simulink model "Electrochmical_simulink"  (R2022a)
settings: Solver=VariableStepAuto  StartTime=0.0  StopTime=10.0  RelTol=1e-3
settings Model: Creator=Anupp  LastModifiedBy=Anupp

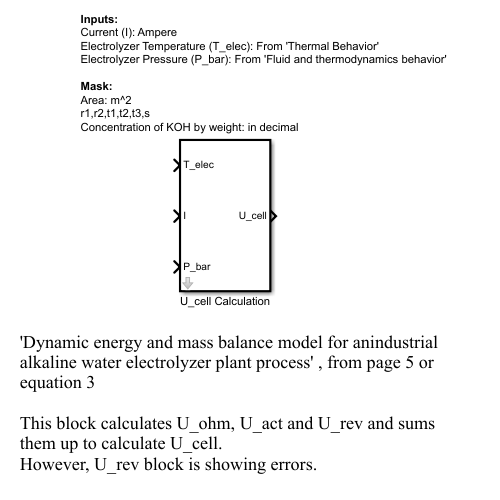
[thumbnail: Simulink's stored preview of the top-level diagram]
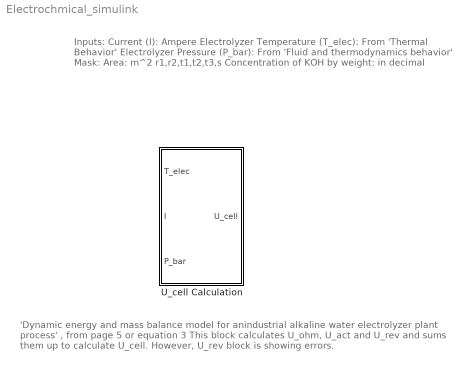
== system Electrochmical_simulink ==
  note: Inputs:
      | Current (I): Ampere
      | Electrolyzer Temperature (T_elec): From 'Thermal Behavior'
      | Electrolyzer Pressure (P_bar): From 'Fluid and thermodynamics behavior'
      |
      | Mask:
      | Area: m^2
      | r1,r2,t1,t2,t3,s
      | Concentration of KOH by weight: in decimal
  note: 'Dynamic energy and mass balance model for anindustrial alkaline water electrolyzer plant process' , from page 5 or equation 3
      |
      | This block calculates U_ohm, U_act and U_rev and sums them up to calculate U_cell.
      | However, U_rev block is showing errors.
  U_cell Calculation : Subsystem  TreatAsAtomicUnit=on  mask{A=0, r1=0, r2=0, t1=0, t2=0, t3=0, s=0, C=0}
      mask prompts: A "Area"; r1 "r1 for U_ohm"; r2 "r2 for U_ohm"; t1 "t1 for U_act"; t2 "t2 for U_act"; t3 "t3 for U_act"; s "s for U_act"; C "Concentration by weight (decimal)"
      mask DialogControl DescTextVar Prompt: Put all values in terms in Metres only or Cm only. Also check if U_act variables is for Log or Ln (change accordingly inside the mask). Also, use concentration value as decimal (for eg. use 0.25, don't use 25 percent).

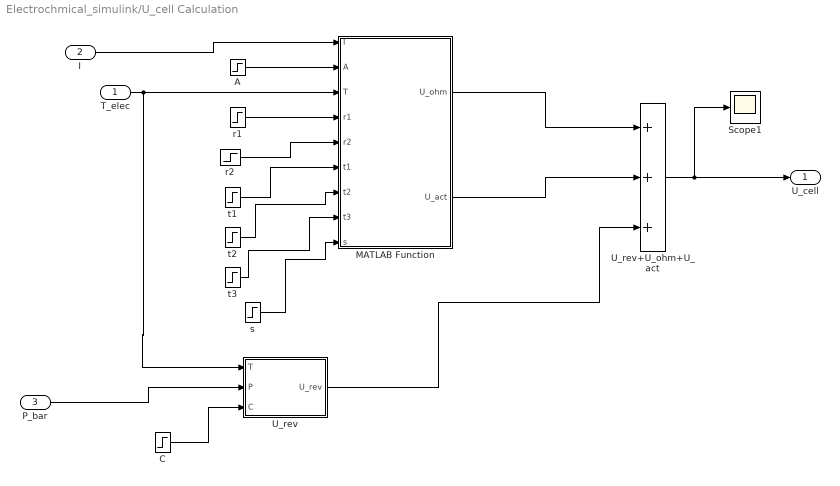
== system Electrochmical_simulink/U_cell Calculation ==
  T_elec : Inport
  I : Inport  Port=2
  P_bar : Inport  Port=3
  A : Step  Time=0  After=A  SampleTime=0
  C : Step  Time=0  After=C  SampleTime=0
  MATLAB Function : MATLAB Function  TreatAsAtomicUnit=on
  Scope1 : Scope
  U_rev : MATLAB Function  TreatAsAtomicUnit=on
  U_rev+U_ohm+U_act : Sum  Inputs=+++
  r1 : Step  Time=0  After=r1  SampleTime=0
  r2 : Step  Time=0  After=r2  SampleTime=0
  s : Step  Time=0  After=s  SampleTime=0
  t1 : Step  Time=0  After=t1  SampleTime=0
  t2 : Step  Time=0  After=t2  SampleTime=0
  t3 : Step  Time=0  After=t3  SampleTime=0
  U_cell : Outport
  wires:
  U_rev/1(U_rev) -> U_rev+U_ohm+U_act/3
  T_elec/1 -> U_rev/1(T), MATLAB Function/3(T)
  P_bar/1 -> U_rev/2(P)
  U_rev+U_ohm+U_act/1 -> U_cell/1, Scope1/1
  C/1 -> U_rev/3(C)
  r1/1 -> MATLAB Function/4(r1)
  r2/1 -> MATLAB Function/5(r2)
  t1/1 -> MATLAB Function/6(t1)
  t2/1 -> MATLAB Function/7(t2)
  t3/1 -> MATLAB Function/8(t3)
  s/1 -> MATLAB Function/9(s)
  I/1 -> MATLAB Function/1(I)
  A/1 -> MATLAB Function/2(A)
  MATLAB Function/2(U_act) -> U_rev+U_ohm+U_act/2
  MATLAB Function/1(U_ohm) -> U_rev+U_ohm+U_act/1

== matlab function Electrochmical_simulink/U_cell Calculation/MATLAB Function ==
  data: I input; U_ohm output; A input; T input; r1 input; r2 input; t1 input; t2 input; t3 input; s input; U_act output
%% Inputs: 
% Current(I): Ampere 
% Area(A): m^2 
% Electrolyzer Temperature(T): K or C (depends on r and t parameters) 
% r1,r2,t1,t2,t3,s: Electrolyzer parameters (Look units carefully)

%% Outputs:
% ohmic voltage loss (U_ohm): V
% Activation voltage loss (U_act): V

%% Main function

function [U_ohm, U_act] = fcn(I,A,T,r1,r2,t1,t2,t3,s)

i = I/A;

U_ohm = (r1 + r2*T)*i;

U_act = s*log((t1 + t2/T + t3/(T^2))*i + 1);

end

== matlab function Electrochmical_simulink/U_cell Calculation/U_rev ==
  data: T input; U_rev output; P input; C input
%% Inputs: 
% Electrolyzer Temperature (T): Kelvin 
% Electrolyzer Pressure(P): bar 
% KOH concentration by weight: in decimal

%% Output: 
% Reversible voltage (U_rev): V

%% Main Function

function U_rev = fcn(T,P,C)
R = 8.3144598; %J. mol-1
z = 2; %of hydrogen is used, don't know why oxygen is not used
F = 96485; %Faradays constant C/mol
M = ((312500/17533)*C)/(1-C); %molality

U_0rev = 1.5184-1.5421*10^(-3)*T+9.526*10^(-5)*T*log(T)+9.84*10^(-8)*(T)^2;

a = -0.0151*M - 1.6788*10^(-3)*(M^2)+2.2588*10^(-5)*(M^3);
b = 1-1.2062*10^(-3)*M+5.6024*10^(-4)*(M^2)-7.8228*10^(-6)*(M^3);
P_vH2O = 10^(5.1962-(1730.63/(233.426+T-273)));
%P_vH2O = exp(81.6179 - 7699.68/T - 10.9*log(T) + 9.5891 * 10^(-3) * T);

P_vKOH = exp(2.302*a+b*log(P_vH2O));

a_H2O_KOH = exp(-0.05192*M+0.003302*(M^2)+((3.177*M-2.131*(M^2))/T));

U_rev = U_0rev + ((R*T)/(z*F))*log(((P-P_vKOH)*((P-P_vKOH)^0.5))/(a_H2O_KOH));

end
